simulink model "CableRobot_2T_preload"  (R2019b)
settings: Solver=ode3  StartTime=0.0  StopTime=tend_sim  FixedStep=stepsize  MaxStep=1e-3  RelTol=1e-3
InitFcn:
  | close all
  | clear
  | Simulink.sdi.clear
  | run scripts\init_model.m
StartFcn:
  | tic
StopFcn:
  | computation_time = toc;
undefined symbols (not defined in the file): Dy0, Y, y0
settings Model: Creator=ac123748  LastModifiedBy=ac123748
settings DataIOCC: SaveOutput=off  ReturnWorkspaceOutputs=off  SignalLoggingName=tmp_raccel_logsout
settings OptimizationCC: EfficientMapNaN2IntZero=off
settings DebuggingCC: ArithmeticOperatorsInVariantConditions=warning
settings HardwareCC: TargetBitPerPointer=64  TargetBitPerSizeT=64  TargetBitPerPtrDiffT=64  TargetLongLongMode=on  TargetIntDivRoundTo=Zero  TargetEndianess=LittleEndian  TargetWordSize=64  TargetHWDeviceType=MATLAB Host  ProdEqTarget=off
settings SFSimCC: SimUseLocalCustomCode=off  CustomCodeUndefinedFunction=UseInterfaceOnly
settings RTWCC: SystemTargetFile=raccel.tlc  TemplateMakefile=raccel_default_tmf  RTWVerbose=off  RTWUseLocalCustomCode=off  RTWUseSimCustomCode=on
settings CodeAppCC: GenerateComments=off  MaxIdLength=128  SimulinkBlockComments=off
settings RaccelTargetCC: GeneratePreprocessorConditionals=Use local settings  LogVarNameModifier=rt_  MultiInstanceERTCode=off  PreserveStateflowLocalDataDimensions=off  ENABLE_SLEXEC_SSBRIDGE=0  RTWCAPISignals=off  RTWCAPIParams=off

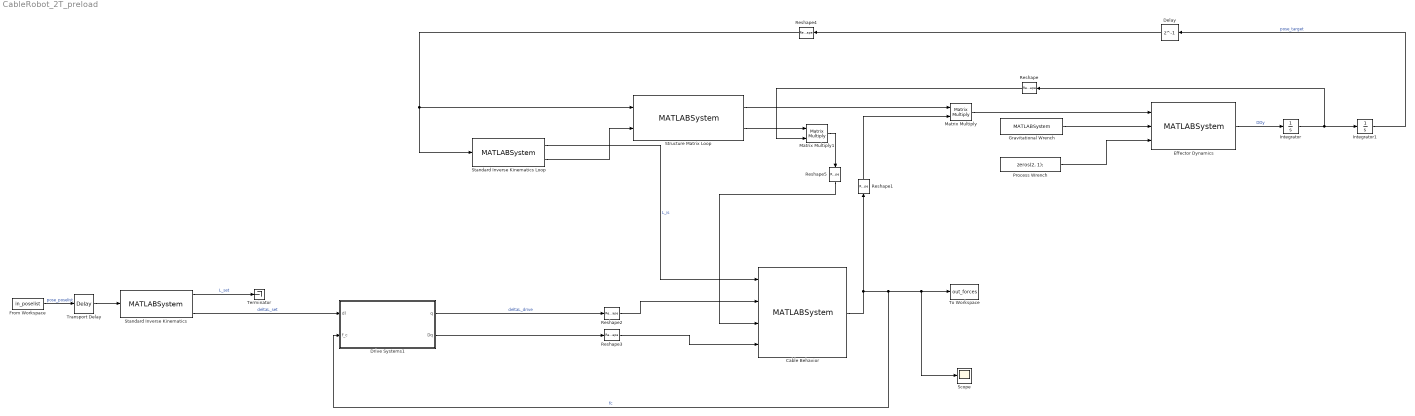
== system CableRobot_2T_preload ==
  Cable Behavior : MATLABSystem  System=cable.linearelasticity  Elasticity=k_elast  Viscosity=d_damp  Reference_Length=Cable_ReferenceLength  Initial_Length=Cable_InitialLength  Model=spring-damper  SimulateUsing=Interpreted execution
      mask Type: cable.linearelasticity
      mask Display:
      | disp(['2T' char(10) 'Cable Dynamics' char(10) 'Linear Elasticity']);
      | port_label('input',1,'l');
      | port_label('input',2,'q');
      | port_label('input',3,'Dl');
      | port_label('input',4,'Dq');
      | port_label('output',1,'fc');
  Delay : Delay  DelayLength=1
  Drive Systems1 : Subsystem
  Effector Dynamics : MATLABSystem  System=dynamics.platform  Weight=PlatformWeight  SimulateUsing=Code generation
      mask Type: dynamics.platform
      mask Display:
      | disp(['2T' char(10) 'Platform Dynamics']);
      | port_label('input',1,'wc');
      | port_label('input',2,'wg');
      | port_label('input',3,'wp');
      | port_label('output',1,'DDy');
  From Workspace : FromWorkspace  VariableName=in_poselist  SampleTime=0
  Gravitational Wrench : MATLABSystem  System=dynamics.gravity  Gravity=9.81  Weight=PlatformWeight  Direction=Y-  SimulateUsing=Code generation
      mask Type: dynamics.gravity
      mask Display:
      | disp(['2T' char(10) 'Gravitational Wrench']);
      | port_label('output',1,'wg');
  Integrator : Integrator  InitialCondition=Dy0
  Integrator1 : Integrator  InitialCondition=y0
  Matrix Multiply : Product  Multiplication=Matrix(*)
  Matrix Multiply1 : Product  Multiplication=Matrix(*)
  Process Wrench : Constant  Value=zeros(2, 1);  VectorParams1D=off
  Reshape : Reshape  OutputDimensionality=Column vector (2-D)
  Reshape1 : Reshape  OutputDimensionality=Column vector (2-D)
  Reshape2 : Reshape  OutputDimensionality=Row vector (2-D)
  Reshape3 : Reshape  OutputDimensionality=Row vector (2-D)
  Reshape4 : Reshape  OutputDimensionality=Column vector (2-D)
  Reshape5 : Reshape  OutputDimensionality=Row vector (2-D)
  Scope : Scope
  Standard Inverse Kinematics : MATLABSystem  System=ik.standard  UnitVectors=on  PulleyAngles=off  DeltaLength=on  MotionPattern=2T  Frame=FrameAnchors  Platform=zeros( 3, 1 )  InitialPose=zeros( 1, 2 )  CableOffset=Cable_Offset
      mask Type: ik.standard
      mask Display:
      | disp('ik.standard');
      | port_label('input',1,'p');
      | port_label('output',1,'l');
      | port_label('output',2,'u');
      | port_label('output',3,'dl');
  Standard Inverse Kinematics Loop : MATLABSystem  System=ik.standard  UnitVectors=on  PulleyAngles=off  DeltaLength=off  MotionPattern=2T  Frame=FrameAnchors  Platform=zeros( 3, 1 )  InitialPose=zeros( 1, 2 )  CableOffset=Cable_Offset
      mask Type: ik.standard
      mask Display:
      | disp('ik.standard');
      | port_label('input',1,'p');
      | port_label('output',1,'l');
      | port_label('output',2,'u');
  Structure Matrix Loop : MATLABSystem  System=sm.structurematrix  Jacobian=on  Nullspace=off  MotionPattern=2T  Platform=zeros( 3, 1 )
      mask Type: sm.structurematrix
      mask Display:
      | disp('sm.structurematrix');
      | port_label('input',1,'p');
      | port_label('input',2,'u');
      | port_label('output',1,'At');
      | port_label('output',2,'J');
  Terminator : Terminator
  To Workspace : ToWorkspace  VariableName=out_forces  SaveFormat=Structure With Time  SampleTime=-1
  Transport Delay : TransportDelay
  wires:
  From Workspace/1 -> Transport Delay/1  "pose_poselist"
  Effector Dynamics/1 -> Integrator/1  "DDy"
  Structure Matrix Loop/1 -> Matrix Multiply/1
  Structure Matrix Loop/2 -> Matrix Multiply1/1
  Standard Inverse Kinematics/1 -> Terminator/1  "L_set"
  Standard Inverse Kinematics Loop/2 -> Structure Matrix Loop/2
  Integrator1/1 -> Delay/1  "pose_target"
  Cable Behavior/1 -> Reshape1/1, Drive Systems1/2(f_c), Scope/1, To Workspace/1  "fc"
  Integrator/1 -> Reshape/1, Integrator1/1
  Standard Inverse Kinematics/3 -> Drive Systems1/1(dl)  "deltaL_set"
  Process Wrench/1 -> Effector Dynamics/3
  Matrix Multiply/1 -> Effector Dynamics/1
  Gravitational Wrench/1 -> Effector Dynamics/2
  Reshape/1 -> Matrix Multiply1/2
  Standard Inverse Kinematics Loop/1 -> Cable Behavior/1  "L_is"
  Drive Systems1/1(q) -> Reshape2/1  "deltaL_drive"
  Drive Systems1/2(Dq) -> Reshape3/1
  Transport Delay/1 -> Standard Inverse Kinematics/1
  Reshape2/1 -> Cable Behavior/2
  Reshape3/1 -> Cable Behavior/4
  Matrix Multiply1/1 -> Reshape5/1
  Reshape1/1 -> Matrix Multiply/2
  Reshape4/1 -> Standard Inverse Kinematics Loop/1, Structure Matrix Loop/1
  Reshape5/1 -> Cable Behavior/3
  Delay/1 -> Reshape4/1

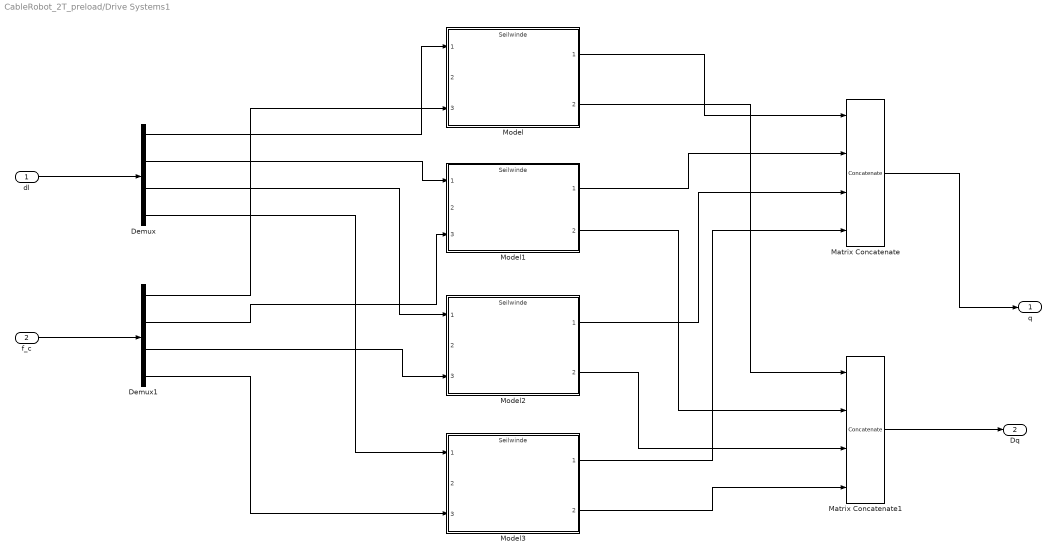
== system CableRobot_2T_preload/Drive Systems1 ==
  dl : Inport
  f_c : Inport  Port=2
  Demux : Demux
  Demux1 : Demux
  Matrix Concatenate : Concatenate  NumInputs=4  ConcatenateDimension=2
  Matrix Concatenate1 : Concatenate  NumInputs=4  ConcatenateDimension=2
  Model{,1..3} (4 alike) : ModelReference  ModelNameDialog=Seilwinde.slx  SimulationMode=Normal  ModelReferenceVersion=1.52
  q : Outport  VectorParamsAs1DForOutWhenUnconnected=off
  Dq : Outport  Port=2  VectorParamsAs1DForOutWhenUnconnected=off
  wires:
  dl/1 -> Demux/1
  Matrix Concatenate/1 -> q/1
  Matrix Concatenate1/1 -> Dq/1
  Demux/2 -> Model1/1
  Demux/3 -> Model2/1
  Demux/4 -> Model3/1
  Model1/1 -> Matrix Concatenate/2
  Model2/1 -> Matrix Concatenate/3
  Model3/1 -> Matrix Concatenate/4
  Model1/2 -> Matrix Concatenate1/2
  Model2/2 -> Matrix Concatenate1/3
  Model3/2 -> Matrix Concatenate1/4
  f_c/1 -> Demux1/1
  Demux/1 -> Model/1
  Model/1 -> Matrix Concatenate/1
  Model/2 -> Matrix Concatenate1/1
  Demux1/1 -> Model/3
  Demux1/2 -> Model1/3
  Demux1/3 -> Model2/3
  Demux1/4 -> Model3/3
